simulink model "quaterrorsim"  (R2017a)
settings: Solver=VariableStepAuto  StartTime=0.0  StopTime=10  RelTol=1e-3
libraries: dspmtrx3 x4, aerolibutil x2
settings Model: Creator=pc  LastModifiedBy=pc

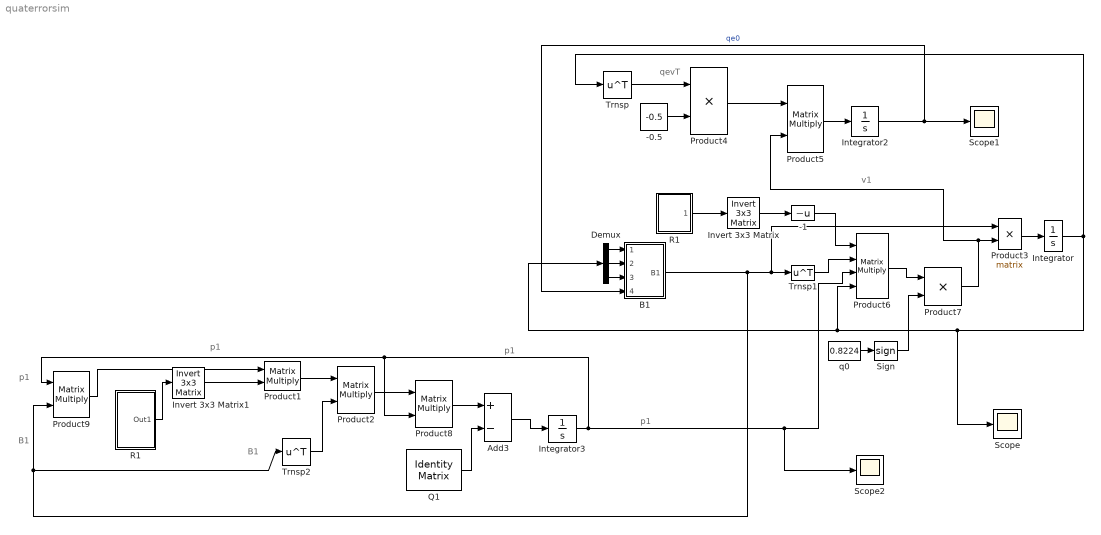
== system quaterrorsim ==
  note: v1
  note: p1
  note: B1
  note: p1
  note: B1
  note: p1
  note: p1
  note: qevT
  -0.5 : Constant  Value=-0.5
  -1 : UnaryMinus
  Add3 : Sum  Inputs=+-
  B1 : Subsystem
  Demux : Demux  Outputs=3
  Integrator : Integrator  InitialCondition=[0.226 0.4397 0.3604]
  Integrator2 : Integrator  InitialCondition=0.8224
  Integrator3 : Integrator  InitialCondition=zeros(3,3)
  Invert 3x3 Matrix : aerolibutil/Invert  3x3 Matrix
  Invert 3x3 Matrix1 : aerolibutil/Invert  3x3 Matrix
  Product{1..3,5,8..9} (6 alike) : Product  Multiplication=Matrix(*)
  Product4 : Product
  Product6 : Product  Inputs=4  Multiplication=Matrix(*)
  Product7 : Product
  Q1 : dspmtrx3/Identity Matrix  Inherit=off  N=3  Ts=1  dataType=double  isSigned=on  wordLen=16  udDataType=sfix(16)  fracBitsMode=Best precision  numFracBits=15  OutDataTypeStr=double  LastOutDataTypeStr=double
      settings: SourceProductName=DSP System Toolbox
  R1 : Subsystem
  "R1 " : Subsystem
  Scope : Scope
  Scope1 : Scope
  Scope2 : Scope
  Sign : Signum
  Trnsp : Math  Operator=transpose  SaturateOnIntegerOverflow=on
  Trnsp1 : Math  Operator=transpose  SaturateOnIntegerOverflow=on
  Trnsp2 : Math  Operator=transpose  SaturateOnIntegerOverflow=on
  q0 : Constant  Value=0.8224
  wires:
  Integrator3/1 -> Product8/2, Product9/1, Scope2/1, Product6/3
  R1/1(Out1) -> Invert 3x3 Matrix/1
  Invert 3x3 Matrix/1 -> -1/1
  q0/1 -> Sign/1
  Product6/1 -> Product7/1
  Sign/1 -> Product7/2
  Product9/1 -> Product1/1
  B1/1(B1) -> Product9/2, Trnsp2/1, Product3/1, Trnsp1/1
  "R1 "/1(Out1) -> Invert 3x3 Matrix1/1
  Product1/1 -> Product2/1
  Trnsp2/1 -> Product2/2
  Q1/1 -> Add3/2
  Invert 3x3 Matrix1/1 -> Product1/2
  Product2/1 -> Product8/1
  Add3/1 -> Integrator3/1
  Product8/1 -> Add3/1
  -1/1 -> Product6/1
  Trnsp1/1 -> Product6/2
  Product3/1 -> Integrator/1
  Product4/1 -> Product5/1
  Trnsp/1 -> Product4/1
  Product5/1 -> Integrator2/1
  Integrator/1 -> Scope/1, Product6/4, Demux/1, Trnsp/1
  -0.5/1 -> Product4/2
  Product7/1 -> Product5/2, Product3/2
  Integrator2/1 -> Scope1/1, B1/4(qe0)  "qe0"
  Demux/1 -> B1/1(qe1)
  Demux/2 -> B1/2(qe2)
  Demux/3 -> B1/3(qe3)

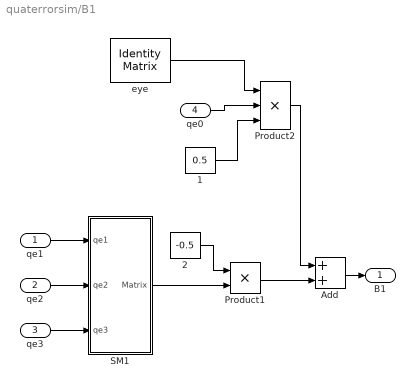
== system quaterrorsim/B1 ==
  qe1 : Inport  PortDimensions=1
  qe2 : Inport  Port=2  PortDimensions=1
  qe3 : Inport  Port=3  PortDimensions=1
  qe0 : Inport  Port=4  PortDimensions=1
  1 : Constant  Value=0.5
  2 : Constant  Value=-0.5
  Add : Sum
  Product1 : Product
  Product2 : Product  Inputs=3
  SM1 : Subsystem
  eye : dspmtrx3/Identity Matrix  Inherit=off  N=3  Ts=1  dataType=double  isSigned=on  wordLen=16  udDataType=sfix(16)  fracBitsMode=Best precision  numFracBits=15  OutDataTypeStr=double  LastOutDataTypeStr=double
      settings: SourceProductName=DSP System Toolbox
  B1 : Outport
  wires:
  Add/1 -> B1/1
  Product2/1 -> Add/1
  SM1/1(Matrix) -> Product1/2
  qe1/1 -> SM1/1(qe1)
  qe2/1 -> SM1/2(qe2)
  eye/1 -> Product2/1
  Product1/1 -> Add/2
  2/1 -> Product1/1
  qe0/1 -> Product2/2
  qe3/1 -> SM1/3(qe3)
  1/1 -> Product2/3

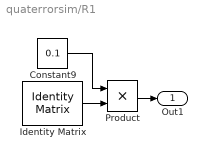
== system quaterrorsim/R1 ==
  Constant9 : Constant  Value=0.1
  Identity Matrix : dspmtrx3/Identity Matrix  Inherit=off  N=3  Ts=1  dataType=double  isSigned=on  wordLen=16  udDataType=sfix(16)  fracBitsMode=Best precision  numFracBits=15  OutDataTypeStr=double  LastOutDataTypeStr=double
      settings: SourceProductName=DSP System Toolbox
  Product : Product
  Out1 : Outport
  wires:
  Identity Matrix/1 -> Product/2
  Constant9/1 -> Product/1
  Product/1 -> Out1/1

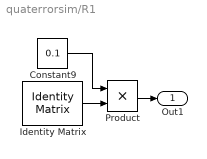
== system quaterrorsim/R1  ==
  Constant9 : Constant  Value=0.1
  Identity Matrix : dspmtrx3/Identity Matrix  Inherit=off  N=3  Ts=1  dataType=double  isSigned=on  wordLen=16  udDataType=sfix(16)  fracBitsMode=Best precision  numFracBits=15  OutDataTypeStr=double  LastOutDataTypeStr=double
      settings: SourceProductName=DSP System Toolbox
  Product : Product
  Out1 : Outport
  wires:
  Identity Matrix/1 -> Product/2
  Constant9/1 -> Product/1
  Product/1 -> Out1/1

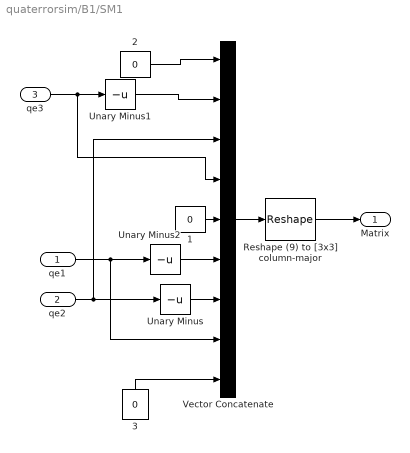
== system quaterrorsim/B1/SM1 ==
  qe1 : Inport  PortDimensions=1
  qe2 : Inport  Port=2  PortDimensions=1
  qe3 : Inport  Port=3  PortDimensions=1
  1 : Constant  Value=0
  2 : Constant  Value=0
  3 : Constant  Value=0
  Reshape (9) to [3x3] column-major : Reshape  OutputDimensionality=Customize  OutputDimensions=[3,3]
  Unary Minus : UnaryMinus
  Unary Minus1 : UnaryMinus
  Unary Minus2 : UnaryMinus
  Vector Concatenate : Concatenate  NumInputs=9
  Matrix : Outport  PortDimensions=[3 3]
  wires:
  qe3/1 -> Unary Minus1/1, Vector Concatenate/4
  Vector Concatenate/1 -> Reshape (9) to [3x3] column-major/1
  Reshape (9) to [3x3] column-major/1 -> Matrix/1
  2/1 -> Vector Concatenate/1
  1/1 -> Vector Concatenate/5
  3/1 -> Vector Concatenate/9
  qe1/1 -> Unary Minus2/1, Vector Concatenate/8
  qe2/1 -> Vector Concatenate/3, Unary Minus/1
  Unary Minus1/1 -> Vector Concatenate/2
  Unary Minus2/1 -> Vector Concatenate/6
  Unary Minus/1 -> Vector Concatenate/7
